simulink model "Electrical_System_2018b_obfs"  (R2019b)
settings: Solver=VariableStepAuto  StartTime=0.0  StopTime=5  RelTol=1e-3  AbsTol=1e-3  EnableMultiTasking=on
InitFcn:
  | Steady_State_Initialisation;
StopFcn:
  | %sscexplore(simlog);
  | %Logging
undefined symbols (not defined in the file): abrlhklxvp, aexgmhuedq, afmfmjnutg, afpphrjpnc, ahuxbyvruc, alarvljztt, amxnyqmnuw, aodrlwvqie, aolhmuplyq, aqpmguuqkg, auesgwirzl, aurophlnng, awamelrhru, ayfhvxflxn, azxkacuhqc, babszerikg, bawhdqanwq, bevoqecvei, bltjvqbchx, bmqsuewujl, bsmyqjfgnf, btvjbsmnve, bywgxqeadw, bziaduxaer, bzmcmdqocb, bzsvyvetat, ccsjnrbsih, cdvenygxwh, cedkrnslhx, cjheorclzs, cjrdshrtqx, ckhavyhcza, ckxewznhlz, cmrcgyiplk, conenicnws, cqkejbgjnn, csfnuwymhe, cunupkhwbh, cwzfvzuxxh, dcadmadufn, dcfponivnv, ddtrqjrhjn, dfhoxvkqas, dfrhtcwpne, dfvomcagjv, djijwylxea, dnmeqksrrm, dnzewbdkaa, dsqcykyxav, dtswwlttmm, ecumpidjtv, edegaywrct, ejjjsmnejc, eknqnehjdz, emvdetzouf, esxbqkbahr, etnkkbreiq, eunoiiiirw, ewewcuedir, fatkfxdhtc ... (+386)
libraries: fl_lib x802, ee_lib x362, fl_ps_legacy_lib x160, nesl_utility x85
(part 18 of 26)

== system Electrical_System_2018b_obfs/Redacted_1221/Redacted_7996/Redacted_7418/Redacted_4377/Redacted_6082/Redacted_2799 ==
  Redacted_14 : fl_lib/Electrical/Electrical Elements/Switch  R_closed=mmaagsrgbc Ohm  G_open=cicknjhhvm 1/Ohm  Threshold=xnzgccqlwj  i_specify=off  i_priority=None  i=hqzepkyeei A  i_nominal_specify=off  i_nominal_unit=A  i_nominal_value=vodnpbetmk  v_specify=off  v_priority=None  v=flyaivdfjk V  v_nominal_specify=off  v_nominal_unit=V  v_nominal_value=przswfymwq
      settings: SourceProductName=Simscape
  Redacted_256 : fl_lib/Electrical/Electrical Elements/Switch  R_closed=ppwmazeqls Ohm  G_open=zeylpmfzmb 1/Ohm  Threshold=xmbikwqmhm  i_specify=off  i_priority=None  i=ajinaowkbj A  i_nominal_specify=off  i_nominal_unit=A  i_nominal_value=uuuzewolju  v_specify=off  v_priority=None  v=otrqqffjwk V  v_nominal_specify=off  v_nominal_unit=V  v_nominal_value=zwxonvfcbj
      settings: SourceProductName=Simscape
  Redacted_3742 : ee_lib/Passive/Thermal/Thermal Resistor  R=xzmplidnqf K/W  T_specify=off  T_priority=None  T=zshsvjmvwr K  T_nominal_specify=off  T_nominal_unit=K  T_nominal_value=dosrqiwvts  Q_specify=off  Q_priority=None  Q=vqlgxiumlf W  Q_nominal_specify=off  Q_nominal_unit=W  Q_nominal_value=mzjjyrayck
      settings: SourceProductName=Simscape Electrical  SourceProductBaseCode=PS  InternalSimscapePortConfiguration="{\"Bottom\":[],\"Left\":[{\"id\":\"A\",\"label\":\"A\",\"type\":\"foundation.thermal.thermal\"}],\"Right\":[{\"id\":\"B\",\"label\":\"B\",\"type\":\"foundation.thermal.thermal\"}],\"Top\":[]}"
  Redacted_4034 : ee_lib/Passive/Thermal/Thermal Resistor  R=xwkozwvuwb K/W  T_specify=off  T_priority=None  T=hxycofyxfo K  T_nominal_specify=off  T_nominal_unit=K  T_nominal_value=yypnighnae  Q_specify=off  Q_priority=None  Q=mmafkkrzqa W  Q_nominal_specify=off  Q_nominal_unit=W  Q_nominal_value=whndbctdlx
      settings: SourceProductName=Simscape Electrical  SourceProductBaseCode=PS  InternalSimscapePortConfiguration="{\"Bottom\":[],\"Left\":[{\"id\":\"A\",\"label\":\"A\",\"type\":\"foundation.thermal.thermal\"}],\"Right\":[{\"id\":\"B\",\"label\":\"B\",\"type\":\"foundation.thermal.thermal\"}],\"Top\":[]}"
  Redacted_4173 : ee_lib/Semiconductors & Converters/Diode  ModelType=tulmihwegb  Vf=dqomejmcdo V  Ron=wefygixenj Ohm  Goff=cqmqzxrucq S  prmExp=eiicyzsqpu  I12=ayxwizdrlh A  V12=yndzldaqag V  IS=swswswzyjd A  ec=ortvifamwx  I1=xnvlgvzazo A  V1=cbnxrsibxn V  RS=zfzslnafvj Ohm  Tmeas=srzeczzhrz degC  N_series=cwyeowwnyg  N_parallel=rzzndodaag  Rz=tmlorzgljf Ohm  BV=fcdpsvgqfz V  C_param=oxxhjpqmkx  CJ=xdhdpetjne pF  CJ0=eopnboxorm pF  VJ=osjqldaapg V  Mgrad=sntnlkitgv  Vvec=vvvsqyjwlq V  Cvec=faidvknuuq pF  FC=nuslxbnegp  Q_param=wpcsrdqkcn  iRM=epgeeezymy A  iF=qkvtlopthh A  didt=yhywaaqkgu A/us  trr_factor=qlxokqlwik  trr=cfxrlwsbqd ns  Qrr=kjhgrlkgfn s*uA  TT=bdveackwqn ns  tau=qgwpqgtevn ns  T_param=qqwmufuloj  IS_T2=vwhbwynzbb A  I1_T2=ugrcgywvxl A  V1_T2=ofimnalxnp V  Tmeas2=efpyefnltl degC  EG_param=gkihstmgwh  EG=vfradqqcre eV  XTI_param=azeiyqzslh  XTI=jnhjlssjor  dBVdT=ozrkunrvqi V/K  Tdevice=gcqsygldcg degC  i_specify=off  i_priority=None  i=yclnvvlwuv A  i_nominal_specify=off  i_nominal_unit=A  i_nominal_value=eroqkrkcly  v_specify=off  v_priority=None  v=sctiisahnx V  v_nominal_specify=off  v_nominal_unit=V  v_nominal_value=ussldzyupi  i_capacitor_specify=off  i_capacitor_priority=None  i_capacitor=adyhzwaero A  i_capacitor_nominal_specify=off  i_capacitor_nominal_unit=A  i_capacitor_nominal_value=jlugygwjih  v_capacitor_specify=off  v_capacitor_priority=None  v_capacitor=uxlkbyjunk V  v_capacitor_nominal_specify=off  v_capacitor_nominal_unit=V  v_capacitor_nominal_value=zhqwudjppl  power_dissipated_specify=off  power_dissipated_priority=None  power_dissipated=eibromriex W  power_dissipated_nominal_specify=off  power_dissipated_nominal_unit=W  power_dissipated_nominal_value=juxdnssqlz  thermal_network_parameterization=gnvkpcxwlv  Rth=ihxwbqdmwa K/W  Rth_Foster=beymoszazb K/W  thermal_mass_parameterization=bygkjedpev  thermal_mass=rnhkfesbtn J/K  thermal_mass_Foster=zkazddkcub J/K  thermal_time_constant=iaakoydqnw s  thermal_time_constant_Foster=zdtgarfcaf s  thermal_mass_initial_temperatures=ruibdayvoi degC
      settings: SourceProductName=Simscape Electrical  InternalSimscapePortConfiguration="{\"Bottom\":[],\"Left\":[{\"id\":\"p\",\"label\":\"\",\"type\":\"foundation.electrical.electrical\"},{\"id\":\"H\",\"label\":\"H\",\"type\":\"foundation.thermal.thermal\"}],\"Right\":[{\"id\":\"n\",\"label\":\"\",\"type\":\"foundation.electrical.electrical\"}],\"Top\":[]}"
  Redacted_50 : ee_lib/Semiconductors & Converters/Diode  ModelType=tlslewfaay  Vf=peujyhvzuc V  Ron=iinywwhiso Ohm  Goff=lbfktfkkrr S  prmExp=svcvswqzek  I12=pknawufhfo A  V12=ptfuvbychd V  IS=kjqfnojdfy A  ec=flctrxnrxr  I1=ajwjiqbsyg A  V1=dxtuezywhb V  RS=ulheemthex Ohm  Tmeas=sovotrzsqy degC  N_series=kqfrjgkdxt  N_parallel=dhsfhjofpz  Rz=xnzdbvfipb Ohm  BV=kttennmtew V  C_param=trkauaxxgo  CJ=qjuoxphjll pF  CJ0=opijhorsqm pF  VJ=azylszyafb V  Mgrad=fejdgnaumo  Vvec=djwbizfuud V  Cvec=evrqxahnvx pF  FC=yrjvkpzstx  Q_param=stalshewbg  iRM=wudiijvfdv A  iF=nqxlcedqfp A  didt=lntrihncyz A/us  trr_factor=fttzoyjfdv  trr=smhwpttsrx ns  Qrr=ydzomidzbs s*uA  TT=hjyfmfchst ns  tau=enzaztgnrs ns  T_param=gtoiihraka  IS_T2=wgpmdxanuh A  I1_T2=taohkjiidl A  V1_T2=npstajglku V  Tmeas2=jdqghdjeem degC  EG_param=xydbowopwk  EG=eklyxpehqx eV  XTI_param=rffpudgvve  XTI=tirunttxyy  dBVdT=yhduoargvg V/K  Tdevice=gtbwypmaiu degC  i_specify=off  i_priority=None  i=muiumfxgrk A  i_nominal_specify=off  i_nominal_unit=A  i_nominal_value=rjdhepavsq  v_specify=off  v_priority=None  v=keyakrzcyf V  v_nominal_specify=off  v_nominal_unit=V  v_nominal_value=mwcpixjzyg  i_capacitor_specify=off  i_capacitor_priority=None  i_capacitor=qotnunkrph A  i_capacitor_nominal_specify=off  i_capacitor_nominal_unit=A  i_capacitor_nominal_value=gzchpazxzl  v_capacitor_specify=off  v_capacitor_priority=None  v_capacitor=eabcrxaphd V  v_capacitor_nominal_specify=off  v_capacitor_nominal_unit=V  v_capacitor_nominal_value=nssgdlqfnr  power_dissipated_specify=off  power_dissipated_priority=None  power_dissipated=kfsjsdylea W  power_dissipated_nominal_specify=off  power_dissipated_nominal_unit=W  power_dissipated_nominal_value=wnkkrbgvrf  thermal_network_parameterization=gawhesamhy  Rth=raeaeqquga K/W  Rth_Foster=ekchdoiazc K/W  thermal_mass_parameterization=yketfhwoay  thermal_mass=kizpyrkmou J/K  thermal_mass_Foster=noigqejeeh J/K  thermal_time_constant=klaivuzsnk s  thermal_time_constant_Foster=wylcbbwvso s  thermal_mass_initial_temperatures=meuehfpoun degC
      settings: SourceProductName=Simscape Electrical  InternalSimscapePortConfiguration="{\"Bottom\":[],\"Left\":[{\"id\":\"p\",\"label\":\"\",\"type\":\"foundation.electrical.electrical\"},{\"id\":\"H\",\"label\":\"H\",\"type\":\"foundation.thermal.thermal\"}],\"Right\":[{\"id\":\"n\",\"label\":\"\",\"type\":\"foundation.electrical.electrical\"}],\"Top\":[]}"
  Redacted_5032 : fl_lib/Electrical/Electrical Elements/Switch  R_closed=djyuvtcnkf Ohm  G_open=ejggmgjquq 1/Ohm  Threshold=rlxsobzzrp  i_specify=off  i_priority=None  i=vxccvsshfr A  i_nominal_specify=off  i_nominal_unit=A  i_nominal_value=ztoxdgmkab  v_specify=off  v_priority=None  v=mvnjgiecut V  v_nominal_specify=off  v_nominal_unit=V  v_nominal_value=fpxnpgloww
      settings: SourceProductName=Simscape
  Redacted_6997 : ee_lib/Passive/Thermal/Thermal Resistor  R=azxkacuhqc K/W  T_specify=off  T_priority=None  T=iqpeqfrrvo K  T_nominal_specify=off  T_nominal_unit=K  T_nominal_value=kewkgutqyk  Q_specify=off  Q_priority=None  Q=xgacttlsfx W  Q_nominal_specify=off  Q_nominal_unit=W  Q_nominal_value=yrupjjmulu
      settings: SourceProductName=Simscape Electrical  SourceProductBaseCode=PS  InternalSimscapePortConfiguration="{\"Bottom\":[],\"Left\":[{\"id\":\"A\",\"label\":\"A\",\"type\":\"foundation.thermal.thermal\"}],\"Right\":[{\"id\":\"B\",\"label\":\"B\",\"type\":\"foundation.thermal.thermal\"}],\"Top\":[]}"
  Redacted_7122 : ee_lib/Passive/Thermal/Thermal Resistor  R=gequosakke K/W  T_specify=off  T_priority=None  T=yveprcfpax K  T_nominal_specify=off  T_nominal_unit=K  T_nominal_value=vzsojcelwy  Q_specify=off  Q_priority=None  Q=jkflhtqewf W  Q_nominal_specify=off  Q_nominal_unit=W  Q_nominal_value=faocaagqnm
      settings: SourceProductName=Simscape Electrical  SourceProductBaseCode=PS  InternalSimscapePortConfiguration="{\"Bottom\":[],\"Left\":[{\"id\":\"A\",\"label\":\"A\",\"type\":\"foundation.thermal.thermal\"}],\"Right\":[{\"id\":\"B\",\"label\":\"B\",\"type\":\"foundation.thermal.thermal\"}],\"Top\":[]}"
  Redacted_718 : ee_lib/Semiconductors & Converters/Diode  ModelType=hzwalpwpdj  Vf=crtqorbrdf V  Ron=dtuaqqqqfe Ohm  Goff=ssskqvgjwx S  prmExp=rbylebavah  I12=gbcjlilwdj A  V12=owdgltcsjq V  IS=nrrmnrcxhi A  ec=sjfrliwacd  I1=ovljdrbuka A  V1=yrcvmuinuy V  RS=nwffojunvq Ohm  Tmeas=yszihgrhjc degC  N_series=ztkzvvauwc  N_parallel=yvkmyxeqrq  Rz=kkiditdcii Ohm  BV=eaknkoqwmh V  C_param=foimocfbtl  CJ=eiydzmpinc pF  CJ0=mcraqkkuzs pF  VJ=qixoqbkvst V  Mgrad=hddpjyowgv  Vvec=guheqtzurh V  Cvec=kdhksuhaik pF  FC=zxtvmvrhvb  Q_param=fmikkvhfee  iRM=ezawdmxmlz A  iF=gaopzjixqb A  didt=hjkdhyvheh A/us  trr_factor=zvbgvgmece  trr=ztladfgbbr ns  Qrr=ohghveggkt s*uA  TT=lfuileimpg ns  tau=toqwscqzcc ns  T_param=svdrsfxyhd  IS_T2=fcoybgbwvg A  I1_T2=aovrifrckl A  V1_T2=troutbqqfh V  Tmeas2=dvigyfmojm degC  EG_param=cxgsnvltrw  EG=roaclctwok eV  XTI_param=ytrguanjdf  XTI=oldetdbykz  dBVdT=ldyqodwnbm V/K  Tdevice=icnmseucpq degC  i_specify=off  i_priority=None  i=krxbgvsmwo A  i_nominal_specify=off  i_nominal_unit=A  i_nominal_value=gdoveeisns  v_specify=off  v_priority=None  v=blpovjuhzh V  v_nominal_specify=off  v_nominal_unit=V  v_nominal_value=qhvsoswlfe  i_capacitor_specify=off  i_capacitor_priority=None  i_capacitor=sfqremdvkr A  i_capacitor_nominal_specify=off  i_capacitor_nominal_unit=A  i_capacitor_nominal_value=rbthjluwwx  v_capacitor_specify=off  v_capacitor_priority=None  v_capacitor=gvebduyxks V  v_capacitor_nominal_specify=off  v_capacitor_nominal_unit=V  v_capacitor_nominal_value=fjsbamdorq  power_dissipated_specify=off  power_dissipated_priority=None  power_dissipated=ktvjbeqvqd W  power_dissipated_nominal_specify=off  power_dissipated_nominal_unit=W  power_dissipated_nominal_value=cyunqnofah  thermal_network_parameterization=lzdjpskjxw  Rth=tumeaafnqm K/W  Rth_Foster=kqaslzygnv K/W  thermal_mass_parameterization=jflyujjaso  thermal_mass=fpaibrkbgh J/K  thermal_mass_Foster=aldyeqrjbc J/K  thermal_time_constant=criblmxzbw s  thermal_time_constant_Foster=xulbsaulbf s  thermal_mass_initial_temperatures=glkvlbqhly degC
      settings: SourceProductName=Simscape Electrical  InternalSimscapePortConfiguration="{\"Bottom\":[],\"Left\":[{\"id\":\"p\",\"label\":\"\",\"type\":\"foundation.electrical.electrical\"},{\"id\":\"H\",\"label\":\"H\",\"type\":\"foundation.thermal.thermal\"}],\"Right\":[{\"id\":\"n\",\"label\":\"\",\"type\":\"foundation.electrical.electrical\"}],\"Top\":[]}"
  Redacted_763 : ee_lib/Semiconductors & Converters/Diode  ModelType=hdctycuzkw  Vf=tjvifnxfuv V  Ron=cnydbqsicp Ohm  Goff=ducaetsmtv S  prmExp=qgbhzhbvzj  I12=pirpzvgjxh A  V12=dkeprjwegx V  IS=elthpplyto A  ec=bvpbkohuyv  I1=oqczivjaob A  V1=pewfscyzrv V  RS=zgtelmnpgz Ohm  Tmeas=gkesqynpca degC  N_series=ihjpnnbzyc  N_parallel=lsvielbegb  Rz=ysgpebshgc Ohm  BV=atzidqevfp V  C_param=vplbhtrmxb  CJ=dvdyqfgpqq pF  CJ0=hftyrpqher pF  VJ=zurufrrrwz V  Mgrad=hvkdrxkshh  Vvec=kxomedtgot V  Cvec=xexhjpbttn pF  FC=gjtifhglrj  Q_param=mwolqugnqg  iRM=pdvcemnafx A  iF=bxrrdaeako A  didt=jneszdjouz A/us  trr_factor=bcagsmvxms  trr=ajbtpbmsxe ns  Qrr=txpyoxjdma s*uA  TT=fsnskeowqu ns  tau=cvinejynxs ns  T_param=mouvaixcwb  IS_T2=fijgahlnnp A  I1_T2=dybchooyle A  V1_T2=dfdjvdimdv V  Tmeas2=cmxztdcxjs degC  EG_param=ticuubgjcs  EG=jgngctnbnn eV  XTI_param=uttsmqjhgd  XTI=atjgiyfovh  dBVdT=inqkiimwec V/K  Tdevice=fnsyksgizi degC  i_specify=off  i_priority=None  i=gmoioopqlw A  i_nominal_specify=off  i_nominal_unit=A  i_nominal_value=xchzsubtdb  v_specify=off  v_priority=None  v=mjkywipror V  v_nominal_specify=off  v_nominal_unit=V  v_nominal_value=fkgekcnpiq  i_capacitor_specify=off  i_capacitor_priority=None  i_capacitor=icabnwcske A  i_capacitor_nominal_specify=off  i_capacitor_nominal_unit=A  i_capacitor_nominal_value=aehltcuqgt  v_capacitor_specify=off  v_capacitor_priority=None  v_capacitor=vipeafkiog V  v_capacitor_nominal_specify=off  v_capacitor_nominal_unit=V  v_capacitor_nominal_value=qnnlzbcipg  power_dissipated_specify=off  power_dissipated_priority=None  power_dissipated=hvjtajjhyi W  power_dissipated_nominal_specify=off  power_dissipated_nominal_unit=W  power_dissipated_nominal_value=nnxgpbwzip  thermal_network_parameterization=cwisxqftsu  Rth=jjddvozwen K/W  Rth_Foster=aghwyaukad K/W  thermal_mass_parameterization=atgudzouir  thermal_mass=vyptloybls J/K  thermal_mass_Foster=orlfbhuaos J/K  thermal_time_constant=crvhtflimy s  thermal_time_constant_Foster=hlgkgupwbd s  thermal_mass_initial_temperatures=frbaaqknpb degC
      settings: SourceProductName=Simscape Electrical  InternalSimscapePortConfiguration="{\"Bottom\":[],\"Left\":[{\"id\":\"p\",\"label\":\"\",\"type\":\"foundation.electrical.electrical\"},{\"id\":\"H\",\"label\":\"H\",\"type\":\"foundation.thermal.thermal\"}],\"Right\":[{\"id\":\"n\",\"label\":\"\",\"type\":\"foundation.electrical.electrical\"}],\"Top\":[]}"
  Redacted_7641 : ee_lib/Semiconductors & Converters/Diode  ModelType=jvmhhockpn  Vf=lzenknmagk V  Ron=amnubdtfvp Ohm  Goff=qakyhwvous S  prmExp=blzattelof  I12=wpanytdecq A  V12=prkwojorfo V  IS=hgjjhzphes A  ec=oewpcqfnkh  I1=vyspsvooxy A  V1=huknxinpvz V  RS=ywhdnctyml Ohm  Tmeas=blplfcoefb degC  N_series=nklolauvfh  N_parallel=ddnyewkblt  Rz=tyiiogmtyz Ohm  BV=agspwlrier V  C_param=mkgmwbzzdz  CJ=drkywxmhpg pF  CJ0=uxzofloada pF  VJ=festuymhqu V  Mgrad=zdmbswzvpp  Vvec=frqpmlhowi V  Cvec=bzftbnihgf pF  FC=nzktvefmus  Q_param=hzlsxtwhka  iRM=tobfsatnwi A  iF=xgehkjzqvu A  didt=wlzrjxtwwo A/us  trr_factor=qmfgsvlxak  trr=uaffhfasez ns  Qrr=vzqlkowmcn s*uA  TT=dtjsuxjcam ns  tau=vqppzywabh ns  T_param=vmteiodvsc  IS_T2=lyxufzuynr A  I1_T2=lbnpebfcgp A  V1_T2=fzfwfrtqhw V  Tmeas2=vcvnwnitjc degC  EG_param=knnbrzbogx  EG=ongjowqasa eV  XTI_param=ukkzrdnnfh  XTI=rtfbrnjfdp  dBVdT=iiiicbmevw V/K  Tdevice=vugruvdnuy degC  i_specify=off  i_priority=None  i=fiocoldtrl A  i_nominal_specify=off  i_nominal_unit=A  i_nominal_value=vdqgzaympr  v_specify=off  v_priority=None  v=wdejrblydg V  v_nominal_specify=off  v_nominal_unit=V  v_nominal_value=tjexfmbrlj  i_capacitor_specify=off  i_capacitor_priority=None  i_capacitor=xlhegmfnlx A  i_capacitor_nominal_specify=off  i_capacitor_nominal_unit=A  i_capacitor_nominal_value=ddhsbhtaaq  v_capacitor_specify=off  v_capacitor_priority=None  v_capacitor=kguleljzqu V  v_capacitor_nominal_specify=off  v_capacitor_nominal_unit=V  v_capacitor_nominal_value=hfthuvzvxo  power_dissipated_specify=off  power_dissipated_priority=None  power_dissipated=hkwkwlmhpj W  power_dissipated_nominal_specify=off  power_dissipated_nominal_unit=W  power_dissipated_nominal_value=orzrmogzgu  thermal_network_parameterization=ovmhndhqct  Rth=ugrkzxpapn K/W  Rth_Foster=ifwzncieyl K/W  thermal_mass_parameterization=laqtytevyp  thermal_mass=zstpknpqqu J/K  thermal_mass_Foster=yuwesjolvn J/K  thermal_time_constant=iubkltnutk s  thermal_time_constant_Foster=gunwrsxdaj s  thermal_mass_initial_temperatures=rdamugqhty degC
      settings: SourceProductName=Simscape Electrical  InternalSimscapePortConfiguration="{\"Bottom\":[],\"Left\":[{\"id\":\"p\",\"label\":\"\",\"type\":\"foundation.electrical.electrical\"},{\"id\":\"H\",\"label\":\"H\",\"type\":\"foundation.thermal.thermal\"}],\"Right\":[{\"id\":\"n\",\"label\":\"\",\"type\":\"foundation.electrical.electrical\"}],\"Top\":[]}"
  Redacted_8838 : ee_lib/Semiconductors & Converters/Diode  ModelType=cmiwftsvec  Vf=vweaeltcps V  Ron=beemewlmho Ohm  Goff=vavlbwhuvj S  prmExp=azknduoumm  I12=nyugqmmbju A  V12=bmiutjqrlm V  IS=bbpownbwtp A  ec=miqmnxjpgq  I1=sxilebsjza A  V1=esprzkqyxr V  RS=tsmillrglu Ohm  Tmeas=giaemdiozw degC  N_series=ryjyzypeuk  N_parallel=vjdnoyxwil  Rz=nxsivwbwly Ohm  BV=jycrnatugz V  C_param=czpybwxoiu  CJ=jncmqgmwwy pF  CJ0=pszifhxfry pF  VJ=muzqxdetft V  Mgrad=jontdzllgi  Vvec=fyabbwyzfg V  Cvec=hkmxdooefi pF  FC=tjdvovdkcd  Q_param=ebwmwlpwww  iRM=nggbgyzjmm A  iF=esjqdcmydr A  didt=vrwzhcrbri A/us  trr_factor=unnpuhacio  trr=rdcmaojzep ns  Qrr=icmuvztiqq s*uA  TT=xzopqsayzy ns  tau=ksscfjmwbz ns  T_param=gczfiuinnw  IS_T2=jfebpqkhnv A  I1_T2=pammjyvwmu A  V1_T2=stdljyyivk V  Tmeas2=cjmrinkojf degC  EG_param=hoqsreszcq  EG=dsrysbmqlv eV  XTI_param=iijwkinkoy  XTI=hmmsrmdojm  dBVdT=bokdbiybpf V/K  Tdevice=dacdhyyaur degC  i_specify=off  i_priority=None  i=zcbvhyriln A  i_nominal_specify=off  i_nominal_unit=A  i_nominal_value=nraaehjrvw  v_specify=off  v_priority=None  v=lcfhjijqqz V  v_nominal_specify=off  v_nominal_unit=V  v_nominal_value=xvhlohnlhz  i_capacitor_specify=off  i_capacitor_priority=None  i_capacitor=zdqctsrrvi A  i_capacitor_nominal_specify=off  i_capacitor_nominal_unit=A  i_capacitor_nominal_value=ttiqqaiibg  v_capacitor_specify=off  v_capacitor_priority=None  v_capacitor=cauazmmjzr V  v_capacitor_nominal_specify=off  v_capacitor_nominal_unit=V  v_capacitor_nominal_value=phzfwhszym  power_dissipated_specify=off  power_dissipated_priority=None  power_dissipated=qurnfxlckn W  power_dissipated_nominal_specify=off  power_dissipated_nominal_unit=W  power_dissipated_nominal_value=ymbbryiklh  thermal_network_parameterization=mmisqbvuit  Rth=glluhycnqd K/W  Rth_Foster=fkkegkuhwv K/W  thermal_mass_parameterization=tcwdmnlntr  thermal_mass=gpzqevvoni J/K  thermal_mass_Foster=opjuznapoq J/K  thermal_time_constant=hmjjgsgsya s  thermal_time_constant_Foster=rghvfyuwvo s  thermal_mass_initial_temperatures=gqkpqornjx degC
      settings: SourceProductName=Simscape Electrical  InternalSimscapePortConfiguration="{\"Bottom\":[],\"Left\":[{\"id\":\"p\",\"label\":\"\",\"type\":\"foundation.electrical.electrical\"},{\"id\":\"H\",\"label\":\"H\",\"type\":\"foundation.thermal.thermal\"}],\"Right\":[{\"id\":\"n\",\"label\":\"\",\"type\":\"foundation.electrical.electrical\"}],\"Top\":[]}"
  Redacted_5480 : PMIOPort  Side=Left
  Redacted_5609 : PMIOPort  Port=2  Side=Left
  Redacted_8475 : PMIOPort  Port=3  Side=Left
  Redacted_2850 : PMIOPort  Port=4  Side=Right
  Redacted_1993 : PMIOPort  Port=5  Side=Right
  Redacted_7871 : PMIOPort  Port=6  Side=Right
  Redacted_7603 : PMIOPort  Port=7  Side=Left
  Redacted_3441 : PMIOPort  Port=8  Side=Right
  connections:
  Redacted_8838/LConn1 -- Redacted_5609/RConn1 -- Redacted_718/RConn1
  Redacted_8838/RConn1 -- Redacted_256/LConn1 -- Redacted_718/LConn1
  Redacted_3742/LConn1 -- Redacted_763/LConn2 -- Redacted_50/LConn2
  Redacted_2850/RConn1 -- Redacted_5032/RConn2
  Redacted_50/LConn1 -- Redacted_5032/LConn1 -- Redacted_763/RConn1
  Redacted_763/LConn1 -- Redacted_5480/RConn1 -- Redacted_50/RConn1
  Redacted_7122/RConn1 -- Redacted_4034/RConn1 -- Redacted_6997/LConn1 -- Redacted_3742/RConn1
  Redacted_7641/LConn1 -- Redacted_8475/RConn1 -- Redacted_4173/RConn1
  Redacted_7871/RConn1 -- Redacted_14/RConn2
  Redacted_3441/RConn1 -- Redacted_14/RConn1 -- Redacted_256/RConn1 -- Redacted_5032/RConn1
  Redacted_1993/RConn1 -- Redacted_256/RConn2
  Redacted_4173/LConn1 -- Redacted_14/LConn1 -- Redacted_7641/RConn1
  Redacted_4173/LConn2 -- Redacted_4034/LConn1 -- Redacted_7641/LConn2
  Redacted_6997/RConn1 -- Redacted_7603/RConn1
  Redacted_8838/LConn2 -- Redacted_718/LConn2 -- Redacted_7122/LConn1

== system Electrical_System_2018b_obfs/Redacted_1221/Redacted_7996/Redacted_7418/Redacted_4377/Redacted_6082/Redacted_2927 ==
  Neutral_Negative : Subsystem  VariantControl=Variant1
  Positive_Neutral : Subsystem  VariantControl=Variant3
  Redacted_9228 : Subsystem  VariantControl=Variant2
  Redacted_7425 : PMIOPort  Side=Left
  Redacted_110 : PMIOPort  Port=2  Side=Left
  Redacted_9932 : PMIOPort  Port=3  Side=Left
  Redacted_5448 : PMIOPort  Port=4  Side=Right
  Redacted_18 : PMIOPort  Port=5  Side=Right

== system Electrical_System_2018b_obfs/Redacted_1221/Redacted_7996/Redacted_7418/Redacted_4377/Redacted_6082/Redacted_3086 ==
  Neutral_Negative : Subsystem  VariantControl=Variant1
  Positive_Neutral : Subsystem  VariantControl=Variant3
  Redacted_7741 : Subsystem  VariantControl=Variant2
  Redacted_6054 : PMIOPort  Side=Left
  Redacted_5626 : PMIOPort  Port=2  Side=Left
  Redacted_6271 : PMIOPort  Port=3  Side=Left
  Redacted_2564 : PMIOPort  Port=4  Side=Right
  Redacted_7933 : PMIOPort  Port=5  Side=Right

== system Electrical_System_2018b_obfs/Redacted_1221/Redacted_7996/Redacted_7418/Redacted_4377/Redacted_6082/Redacted_3181 ==
  Redacted_1351 : ee_lib/Semiconductors & Converters/Diode  ModelType=seeuamuunc  Vf=tjetfrvgds V  Ron=tkwkxekvdq Ohm  Goff=xzxgjjbiog S  prmExp=tjyqkmyyzz  I12=vfldstogen A  V12=aavwtmhros V  IS=bjqywamhpj A  ec=kdkykdyevk  I1=zmbpaboecy A  V1=udzpdlacpc V  RS=jxlihmcwve Ohm  Tmeas=yyfgspfgbd degC  N_series=zsfxqjbunr  N_parallel=fgwiengsno  Rz=avicgvmlgk Ohm  BV=okerteawrl V  C_param=wbkqkuwogq  CJ=wjeiksybxp pF  CJ0=bhyyzfyxjp pF  VJ=baqqiwdxpe V  Mgrad=ijgrywoabh  Vvec=hkmchzqwjs V  Cvec=boveevrcen pF  FC=zabwgjpoen  Q_param=eawnjzzyvy  iRM=kamsrqwhqk A  iF=gaslkmmfnx A  didt=ntyglgoooi A/us  trr_factor=sysuzqibag  trr=yinnobosjz ns  Qrr=jaajtcswbs s*uA  TT=nsneizmgzk ns  tau=gvehbplkpv ns  T_param=rmggrjeyry  IS_T2=bosnjnhbqx A  I1_T2=sevxlylkmu A  V1_T2=kuctfzdxpm V  Tmeas2=xsehdofiyo degC  EG_param=oeofywqxdk  EG=uifethuxrb eV  XTI_param=wtzpwykpco  XTI=jqlhgbjlia  dBVdT=bvciagvedp V/K  Tdevice=wqvmrlhfms degC  i_specify=off  i_priority=None  i=iibbfecdkw A  i_nominal_specify=off  i_nominal_unit=A  i_nominal_value=rqcvvpbxgl  v_specify=off  v_priority=None  v=ozhvdnmemj V  v_nominal_specify=off  v_nominal_unit=V  v_nominal_value=rgrbkwjmip  i_capacitor_specify=off  i_capacitor_priority=None  i_capacitor=hbcekzmgcv A  i_capacitor_nominal_specify=off  i_capacitor_nominal_unit=A  i_capacitor_nominal_value=hspgnyvvck  v_capacitor_specify=off  v_capacitor_priority=None  v_capacitor=ekhmskymom V  v_capacitor_nominal_specify=off  v_capacitor_nominal_unit=V  v_capacitor_nominal_value=kxjlgmioqp  power_dissipated_specify=off  power_dissipated_priority=None  power_dissipated=edojgqvblt W  power_dissipated_nominal_specify=off  power_dissipated_nominal_unit=W  power_dissipated_nominal_value=tsdphnszae  thermal_network_parameterization=asyzzvkyhi  Rth=lywppooubx K/W  Rth_Foster=vecederauj K/W  thermal_mass_parameterization=fsmsxwodxt  thermal_mass=udhbpbteyl J/K  thermal_mass_Foster=kcaieczpfc J/K  thermal_time_constant=qqooakurgg s  thermal_time_constant_Foster=zxqadwzazc s  thermal_mass_initial_temperatures=ljlpeezqox degC
      settings: SourceProductName=Simscape Electrical  InternalSimscapePortConfiguration="{\"Bottom\":[],\"Left\":[{\"id\":\"p\",\"label\":\"\",\"type\":\"foundation.electrical.electrical\"},{\"id\":\"H\",\"label\":\"H\",\"type\":\"foundation.thermal.thermal\"}],\"Right\":[{\"id\":\"n\",\"label\":\"\",\"type\":\"foundation.electrical.electrical\"}],\"Top\":[]}"
  Redacted_3158 : fl_lib/Electrical/Electrical Elements/Switch  R_closed=hwmyltiiqs Ohm  G_open=oageffilii 1/Ohm  Threshold=llxzcykggr  i_specify=off  i_priority=None  i=towpqqbrgr A  i_nominal_specify=off  i_nominal_unit=A  i_nominal_value=yhnwwkhofb  v_specify=off  v_priority=None  v=qsxecyuspm V  v_nominal_specify=off  v_nominal_unit=V  v_nominal_value=iycquvnywo
      settings: SourceProductName=Simscape
  Redacted_3931 : ee_lib/Semiconductors & Converters/Diode  ModelType=tqxwxbyope  Vf=msvpzzkeba V  Ron=fwkchzqblf Ohm  Goff=svlnqffeyd S  prmExp=mlctstspcp  I12=bbyevmnspz A  V12=uvkidbyuvs V  IS=lpydrxcezd A  ec=qsufrycozn  I1=lepjzvxqxl A  V1=ipknupmupx V  RS=bzinarmuqq Ohm  Tmeas=rkwjjzfkwq degC  N_series=imzifmjoup  N_parallel=wbyltkjjsq  Rz=bisuniwcvj Ohm  BV=jgybmonlsf V  C_param=hbgjuibrwj  CJ=gqvyumecto pF  CJ0=ibsphiesxm pF  VJ=bijqmoevpa V  Mgrad=mubmyiximf  Vvec=byiivkqhni V  Cvec=aoibtvakqs pF  FC=copuhvmvyb  Q_param=bflbuobaow  iRM=zldaqxybvj A  iF=ytnymxtjly A  didt=idoehkwwtj A/us  trr_factor=ebltoywncm  trr=fygpxetjfj ns  Qrr=uimcleybda s*uA  TT=krndejyjuq ns  tau=hukxqqjqto ns  T_param=elgqdsktyc  IS_T2=zbjbtcnzao A  I1_T2=hipcbswwjs A  V1_T2=dsoyluttfa V  Tmeas2=fbupxbajck degC  EG_param=mvsexujbus  EG=xiyujyeecx eV  XTI_param=krdlbkxuyu  XTI=xewpkszqxo  dBVdT=ibvfxirjgx V/K  Tdevice=rknouiddqv degC  i_specify=off  i_priority=None  i=ecenxenwrc A  i_nominal_specify=off  i_nominal_unit=A  i_nominal_value=fxilzhobes  v_specify=off  v_priority=None  v=hrmiwxfjsj V  v_nominal_specify=off  v_nominal_unit=V  v_nominal_value=emarxszixz  i_capacitor_specify=off  i_capacitor_priority=None  i_capacitor=febrtrnqtb A  i_capacitor_nominal_specify=off  i_capacitor_nominal_unit=A  i_capacitor_nominal_value=jccfenurhb  v_capacitor_specify=off  v_capacitor_priority=None  v_capacitor=umlvqkknjw V  v_capacitor_nominal_specify=off  v_capacitor_nominal_unit=V  v_capacitor_nominal_value=gghvoucqhq  power_dissipated_specify=off  power_dissipated_priority=None  power_dissipated=amzqicgaia W  power_dissipated_nominal_specify=off  power_dissipated_nominal_unit=W  power_dissipated_nominal_value=oymruehjkf  thermal_network_parameterization=jpsxuylylh  Rth=uehbhvrzjt K/W  Rth_Foster=tejtqvzged K/W  thermal_mass_parameterization=btxpxztosi  thermal_mass=gxhkmzniwp J/K  thermal_mass_Foster=vdvluvqrgk J/K  thermal_time_constant=idwezoowwk s  thermal_time_constant_Foster=iskjzblkee s  thermal_mass_initial_temperatures=rnchfspvkh degC
      settings: SourceProductName=Simscape Electrical  InternalSimscapePortConfiguration="{\"Bottom\":[],\"Left\":[{\"id\":\"p\",\"label\":\"\",\"type\":\"foundation.electrical.electrical\"},{\"id\":\"H\",\"label\":\"H\",\"type\":\"foundation.thermal.thermal\"}],\"Right\":[{\"id\":\"n\",\"label\":\"\",\"type\":\"foundation.electrical.electrical\"}],\"Top\":[]}"
  Redacted_4404 : ee_lib/Passive/Thermal/Thermal Resistor  R=xexuroemqo K/W  T_specify=off  T_priority=None  T=xnbryopseg K  T_nominal_specify=off  T_nominal_unit=K  T_nominal_value=kdpocicxnp  Q_specify=off  Q_priority=None  Q=hdqjdfbsma W  Q_nominal_specify=off  Q_nominal_unit=W  Q_nominal_value=udkikzuzos
      settings: SourceProductName=Simscape Electrical  SourceProductBaseCode=PS  InternalSimscapePortConfiguration="{\"Bottom\":[],\"Left\":[{\"id\":\"A\",\"label\":\"A\",\"type\":\"foundation.thermal.thermal\"}],\"Right\":[{\"id\":\"B\",\"label\":\"B\",\"type\":\"foundation.thermal.thermal\"}],\"Top\":[]}"
  Redacted_6446 : ee_lib/Passive/Thermal/Thermal Resistor  R=hwqngtoeuw K/W  T_specify=off  T_priority=None  T=hsoozjtrph K  T_nominal_specify=off  T_nominal_unit=K  T_nominal_value=dxhlmwnjse  Q_specify=off  Q_priority=None  Q=nagsetwglx W  Q_nominal_specify=off  Q_nominal_unit=W  Q_nominal_value=cxhyvgnbrj
      settings: SourceProductName=Simscape Electrical  SourceProductBaseCode=PS  InternalSimscapePortConfiguration="{\"Bottom\":[],\"Left\":[{\"id\":\"A\",\"label\":\"A\",\"type\":\"foundation.thermal.thermal\"}],\"Right\":[{\"id\":\"B\",\"label\":\"B\",\"type\":\"foundation.thermal.thermal\"}],\"Top\":[]}"
  Redacted_9048 : ee_lib/Passive/Thermal/Thermal Resistor  R=zjtbpuzrue K/W  T_specify=off  T_priority=None  T=etnkkbreiq K  T_nominal_specify=off  T_nominal_unit=K  T_nominal_value=kahcrnokjt  Q_specify=off  Q_priority=None  Q=lionqndkkr W  Q_nominal_specify=off  Q_nominal_unit=W  Q_nominal_value=rkfkvndftj
      settings: SourceProductName=Simscape Electrical  SourceProductBaseCode=PS  InternalSimscapePortConfiguration="{\"Bottom\":[],\"Left\":[{\"id\":\"A\",\"label\":\"A\",\"type\":\"foundation.thermal.thermal\"}],\"Right\":[{\"id\":\"B\",\"label\":\"B\",\"type\":\"foundation.thermal.thermal\"}],\"Top\":[]}"
  Redacted_9733 : fl_lib/Electrical/Electrical Elements/Switch  R_closed=ovhcdwdqkf Ohm  G_open=owpytlrcdh 1/Ohm  Threshold=yzytgmynyn  i_specify=off  i_priority=None  i=owtxshledt A  i_nominal_specify=off  i_nominal_unit=A  i_nominal_value=nybtewbswk  v_specify=off  v_priority=None  v=kpnujakptf V  v_nominal_specify=off  v_nominal_unit=V  v_nominal_value=jucrzeyoqp
      settings: SourceProductName=Simscape
  Redacted_2911 : PMIOPort  Side=Left
  Redacted_7251 : PMIOPort  Port=2  Side=Left
  Redacted_7245 : PMIOPort  Port=3  Side=Right
  Redacted_1415 : PMIOPort  Port=4  Side=Right
  Redacted_532 : PMIOPort  Port=5  Side=Left
  Redacted_2658 : PMIOPort  Port=6  Side=Right
  connections:
  Redacted_3931/LConn1 -- Redacted_7251/RConn1
  Redacted_3931/RConn1 -- Redacted_3158/LConn1
  Redacted_1351/LConn2 -- Redacted_6446/LConn1
  Redacted_7245/RConn1 -- Redacted_9733/RConn2
  Redacted_1351/LConn1 -- Redacted_9733/LConn1
  Redacted_2911/RConn1 -- Redacted_1351/RConn1
  Redacted_4404/RConn1 -- Redacted_9048/LConn1 -- Redacted_6446/RConn1
  Redacted_2658/RConn1 -- Redacted_3158/RConn1 -- Redacted_9733/RConn1
  Redacted_1415/RConn1 -- Redacted_3158/RConn2
  Redacted_9048/RConn1 -- Redacted_532/RConn1
  Redacted_3931/LConn2 -- Redacted_4404/LConn1

== system Electrical_System_2018b_obfs/Redacted_1221/Redacted_7996/Redacted_7418/Redacted_4377/Redacted_6082/Redacted_3818 ==
  Neutral_Negative : Subsystem  VariantControl=Variant1
  Positive_Neutral : Subsystem  VariantControl=Variant3
  Redacted_7647 : Subsystem  VariantControl=Variant2
  Redacted_558 : PMIOPort  Side=Left
  Redacted_9353 : PMIOPort  Port=2  Side=Left
  Redacted_2763 : PMIOPort  Port=3  Side=Left
  Redacted_5509 : PMIOPort  Port=4  Side=Right
  Redacted_3127 : PMIOPort  Port=5  Side=Right

== system Electrical_System_2018b_obfs/Redacted_1221/Redacted_7996/Redacted_7418/Redacted_4377/Redacted_6082/Redacted_4174 ==
  Neutral_Negative : Subsystem  VariantControl=Variant1
  Positive_Neutral : Subsystem  VariantControl=Variant3
  Redacted_8370 : Subsystem  VariantControl=Variant2
  Redacted_9679 : PMIOPort  Side=Left
  Redacted_9878 : PMIOPort  Port=2  Side=Left
  Redacted_224 : PMIOPort  Port=3  Side=Left
  Redacted_5953 : PMIOPort  Port=4  Side=Right
  Redacted_7639 : PMIOPort  Port=5  Side=Right

== system Electrical_System_2018b_obfs/Redacted_1221/Redacted_7996/Redacted_7418/Redacted_4377/Redacted_6082/Redacted_4278 ==
  Neutral_Negative : Subsystem  VariantControl=Variant1
  Positive_Neutral : Subsystem  VariantControl=Variant3
  Redacted_1592 : Subsystem  VariantControl=Variant2
  Redacted_1495 : PMIOPort  Side=Left
  Redacted_2064 : PMIOPort  Port=2  Side=Left
  Redacted_9467 : PMIOPort  Port=3  Side=Left
  Redacted_1543 : PMIOPort  Port=4  Side=Right
  Redacted_9491 : PMIOPort  Port=5  Side=Right

== system Electrical_System_2018b_obfs/Redacted_1221/Redacted_7996/Redacted_7418/Redacted_4377/Redacted_6082/Redacted_4288 ==
  Redacted_1420 : ee_lib/Passive/Thermal/Thermal Resistor  R=csfnuwymhe K/W  T_specify=off  T_priority=None  T=dfrhtcwpne K  T_nominal_specify=off  T_nominal_unit=K  T_nominal_value=undcbzrngw  Q_specify=off  Q_priority=None  Q=qyyvrynvtf W  Q_nominal_specify=off  Q_nominal_unit=W  Q_nominal_value=fykywgxewt
      settings: SourceProductName=Simscape Electrical  SourceProductBaseCode=PS  InternalSimscapePortConfiguration="{\"Bottom\":[],\"Left\":[{\"id\":\"A\",\"label\":\"A\",\"type\":\"foundation.thermal.thermal\"}],\"Right\":[{\"id\":\"B\",\"label\":\"B\",\"type\":\"foundation.thermal.thermal\"}],\"Top\":[]}"
  Redacted_3053 : ee_lib/Passive/Thermal/Thermal Resistor  R=feuklzgtpa K/W  T_specify=off  T_priority=None  T=qwktvjvfys K  T_nominal_specify=off  T_nominal_unit=K  T_nominal_value=arolkdlhmd  Q_specify=off  Q_priority=None  Q=djhelqxest W  Q_nominal_specify=off  Q_nominal_unit=W  Q_nominal_value=dkqmeratgj
      settings: SourceProductName=Simscape Electrical  SourceProductBaseCode=PS  InternalSimscapePortConfiguration="{\"Bottom\":[],\"Left\":[{\"id\":\"A\",\"label\":\"A\",\"type\":\"foundation.thermal.thermal\"}],\"Right\":[{\"id\":\"B\",\"label\":\"B\",\"type\":\"foundation.thermal.thermal\"}],\"Top\":[]}"
  Redacted_5187 : fl_lib/Electrical/Electrical Elements/Switch  R_closed=iidrcmgruo Ohm  G_open=cwflxapbrg 1/Ohm  Threshold=wtaszsnldr  i_specify=off  i_priority=None  i=cfjwrmlajq A  i_nominal_specify=off  i_nominal_unit=A  i_nominal_value=qzidrdxbsm  v_specify=off  v_priority=None  v=hrbzqwpexo V  v_nominal_specify=off  v_nominal_unit=V  v_nominal_value=oarcvjnccc
      settings: SourceProductName=Simscape
  Redacted_5716 : fl_lib/Electrical/Electrical Elements/Switch  R_closed=krkbgwsxlo Ohm  G_open=nwjalbnmwo 1/Ohm  Threshold=wlnjmfizfx  i_specify=off  i_priority=None  i=xtkvqzsayg A  i_nominal_specify=off  i_nominal_unit=A  i_nominal_value=nzimhpxyaj  v_specify=off  v_priority=None  v=dcozybqfae V  v_nominal_specify=off  v_nominal_unit=V  v_nominal_value=cwsubwwopk
      settings: SourceProductName=Simscape
  Redacted_631 : ee_lib/Semiconductors & Converters/Diode  ModelType=kwymznercn  Vf=bzeobnkmpp V  Ron=ogzcuqezum Ohm  Goff=hboakganul S  prmExp=tspwxvmtix  I12=vzhmfidnsx A  V12=lzcdoaedsk V  IS=lxuhqgdzyf A  ec=lgmvvpmtfb  I1=wubgixerlf A  V1=ghqnutyshn V  RS=yfueffmaxl Ohm  Tmeas=ydajfmxqbx degC  N_series=yivbhcvoir  N_parallel=htzntkphxa  Rz=qvvvhxwbpi Ohm  BV=ymjzdmieqs V  C_param=msvgljfcfw  CJ=zsrrieohii pF  CJ0=tuthjrqdnh pF  VJ=nycerhqgyj V  Mgrad=qvizemveid  Vvec=qlenbgnmqk V  Cvec=bligwbbtgp pF  FC=roozurrocc  Q_param=xkglsmbrbh  iRM=qahgubavsm A  iF=pufyexdedl A  didt=isjydruslg A/us  trr_factor=dffqwpsdyp  trr=anfkerbzue ns  Qrr=deomtvnwwe s*uA  TT=lrekwszonl ns  tau=iyastrgkxi ns  T_param=kjwuhembzs  IS_T2=mmckjlxiwy A  I1_T2=llsygjllnm A  V1_T2=ebzpqvnskm V  Tmeas2=dgihdwdint degC  EG_param=vfglbqzjmq  EG=vnjpxdvxmw eV  XTI_param=uocmdbuhnh  XTI=mybmalgdic  dBVdT=fpdhcmbsix V/K  Tdevice=fyegxrufcw degC  i_specify=off  i_priority=None  i=lkokslneyy A  i_nominal_specify=off  i_nominal_unit=A  i_nominal_value=hoeahmmfuu  v_specify=off  v_priority=None  v=jwstxjltpj V  v_nominal_specify=off  v_nominal_unit=V  v_nominal_value=vzfhxnllbc  i_capacitor_specify=off  i_capacitor_priority=None  i_capacitor=myvfxzqlck A  i_capacitor_nominal_specify=off  i_capacitor_nominal_unit=A  i_capacitor_nominal_value=roqvolylnm  v_capacitor_specify=off  v_capacitor_priority=None  v_capacitor=gptluhsrhz V  v_capacitor_nominal_specify=off  v_capacitor_nominal_unit=V  v_capacitor_nominal_value=alzbeepcwm  power_dissipated_specify=off  power_dissipated_priority=None  power_dissipated=uijibnuhos W  power_dissipated_nominal_specify=off  power_dissipated_nominal_unit=W  power_dissipated_nominal_value=lbddeeurpg  thermal_network_parameterization=frunhdzzzq  Rth=ipffswvaig K/W  Rth_Foster=tpgcjeuyzq K/W  thermal_mass_parameterization=jwlodfpkvm  thermal_mass=ehnyrrnqzl J/K  thermal_mass_Foster=unmbisyvtm J/K  thermal_time_constant=oypiywoukf s  thermal_time_constant_Foster=xnmvgxpcww s  thermal_mass_initial_temperatures=zwgjhousxc degC
      settings: SourceProductName=Simscape Electrical  InternalSimscapePortConfiguration="{\"Bottom\":[],\"Left\":[{\"id\":\"p\",\"label\":\"\",\"type\":\"foundation.electrical.electrical\"},{\"id\":\"H\",\"label\":\"H\",\"type\":\"foundation.thermal.thermal\"}],\"Right\":[{\"id\":\"n\",\"label\":\"\",\"type\":\"foundation.electrical.electrical\"}],\"Top\":[]}"
  Redacted_6763 : ee_lib/Semiconductors & Converters/Diode  ModelType=clgixcnwoc  Vf=ftpzcjmppy V  Ron=dbcidwevvn Ohm  Goff=yhrmcwzgue S  prmExp=aisizesfzq  I12=lacnnvocyc A  V12=pbpbsjubgs V  IS=xamdbquppu A  ec=eeecjfdprz  I1=yjljdcozpv A  V1=ffbopghzjw V  RS=wcqnbvzzev Ohm  Tmeas=kbuiibngbo degC  N_series=qqlilfwukw  N_parallel=fxbsiddyro  Rz=dodwndnmkr Ohm  BV=liehghwjmv V  C_param=vktsvahwle  CJ=fhntaxxfft pF  CJ0=qumaznckyu pF  VJ=xpoblmifuo V  Mgrad=ocusdggsnv  Vvec=seffqhedpz V  Cvec=ohcmggolrz pF  FC=yxsxrkinug  Q_param=bvzohlmuww  iRM=xicczpmsfr A  iF=rkcnntyhvb A  didt=vtudfiaipt A/us  trr_factor=rqvaooxfvk  trr=tvwihwyihb ns  Qrr=kulozvhoez s*uA  TT=nitkbtqglp ns  tau=ubqxhynwqh ns  T_param=igxsyorppi  IS_T2=mqvbxmpxvg A  I1_T2=armqecybmn A  V1_T2=muvfioogix V  Tmeas2=ppsjgixytg degC  EG_param=xjxvdcpxwh  EG=agihhvisij eV  XTI_param=yuocwdmjkw  XTI=xoszctygzp  dBVdT=uoohrvaigf V/K  Tdevice=qhfnbogqqg degC  i_specify=off  i_priority=None  i=qtedmgmqsm A  i_nominal_specify=off  i_nominal_unit=A  i_nominal_value=mqkthilpvy  v_specify=off  v_priority=None  v=itpbbundcp V  v_nominal_specify=off  v_nominal_unit=V  v_nominal_value=ykhzflpcnx  i_capacitor_specify=off  i_capacitor_priority=None  i_capacitor=uryfeeajta A  i_capacitor_nominal_specify=off  i_capacitor_nominal_unit=A  i_capacitor_nominal_value=ftxeerromd  v_capacitor_specify=off  v_capacitor_priority=None  v_capacitor=hddhodbyvb V  v_capacitor_nominal_specify=off  v_capacitor_nominal_unit=V  v_capacitor_nominal_value=yzdcvmjrfh  power_dissipated_specify=off  power_dissipated_priority=None  power_dissipated=aaxygncreu W  power_dissipated_nominal_specify=off  power_dissipated_nominal_unit=W  power_dissipated_nominal_value=xuxnetzqve  thermal_network_parameterization=zrkkuhurzb  Rth=odsbqwesbo K/W  Rth_Foster=ibbukupzba K/W  thermal_mass_parameterization=laqxzbiuja  thermal_mass=jqetfysksy J/K  thermal_mass_Foster=rleuvpzybd J/K  thermal_time_constant=vfwhldlplc s  thermal_time_constant_Foster=sredobdxmn s  thermal_mass_initial_temperatures=gkskoiqoer degC
      settings: SourceProductName=Simscape Electrical  InternalSimscapePortConfiguration="{\"Bottom\":[],\"Left\":[{\"id\":\"p\",\"label\":\"\",\"type\":\"foundation.electrical.electrical\"},{\"id\":\"H\",\"label\":\"H\",\"type\":\"foundation.thermal.thermal\"}],\"Right\":[{\"id\":\"n\",\"label\":\"\",\"type\":\"foundation.electrical.electrical\"}],\"Top\":[]}"
  Redacted_938 : ee_lib/Passive/Thermal/Thermal Resistor  R=virfgdrnfz K/W  T_specify=off  T_priority=None  T=alarvljztt K  T_nominal_specify=off  T_nominal_unit=K  T_nominal_value=joqgdgroxe  Q_specify=off  Q_priority=None  Q=kaqfzywiqi W  Q_nominal_specify=off  Q_nominal_unit=W  Q_nominal_value=zlmidgadwg
      settings: SourceProductName=Simscape Electrical  SourceProductBaseCode=PS  InternalSimscapePortConfiguration="{\"Bottom\":[],\"Left\":[{\"id\":\"A\",\"label\":\"A\",\"type\":\"foundation.thermal.thermal\"}],\"Right\":[{\"id\":\"B\",\"label\":\"B\",\"type\":\"foundation.thermal.thermal\"}],\"Top\":[]}"
  Redacted_2382 : PMIOPort  Side=Left
  Redacted_435 : PMIOPort  Port=2  Side=Left
  Redacted_3794 : PMIOPort  Port=3  Side=Right
  Redacted_28 : PMIOPort  Port=4  Side=Right
  Redacted_1383 : PMIOPort  Port=5  Side=Left
  Redacted_1778 : PMIOPort  Port=6  Side=Right
  connections:
  Redacted_6763/LConn1 -- Redacted_435/RConn1
  Redacted_6763/RConn1 -- Redacted_5716/LConn1
  Redacted_631/LConn2 -- Redacted_938/LConn1
  Redacted_3794/RConn1 -- Redacted_5187/RConn2
  Redacted_631/LConn1 -- Redacted_5187/LConn1
  Redacted_2382/RConn1 -- Redacted_631/RConn1
  Redacted_3053/RConn1 -- Redacted_1420/LConn1 -- Redacted_938/RConn1
  Redacted_1778/RConn1 -- Redacted_5716/RConn1 -- Redacted_5187/RConn1
  Redacted_28/RConn1 -- Redacted_5716/RConn2
  Redacted_1420/RConn1 -- Redacted_1383/RConn1
  Redacted_6763/LConn2 -- Redacted_3053/LConn1

== system Electrical_System_2018b_obfs/Redacted_1221/Redacted_7996/Redacted_7418/Redacted_4377/Redacted_6082/Redacted_4413 ==
  Neutral_Negative : Subsystem  VariantControl=Variant1
  Positive_Neutral : Subsystem  VariantControl=Variant3
  Redacted_6190 : Subsystem  VariantControl=Variant2
  Redacted_9976 : PMIOPort  Side=Left
  Redacted_5180 : PMIOPort  Port=2  Side=Left
  Redacted_6712 : PMIOPort  Port=3  Side=Left
  Redacted_6595 : PMIOPort  Port=4  Side=Right
  Redacted_8408 : PMIOPort  Port=5  Side=Right

== system Electrical_System_2018b_obfs/Redacted_1221/Redacted_7996/Redacted_7418/Redacted_4377/Redacted_6082/Redacted_4712 ==
  Redacted_2183 : ee_lib/Passive/Thermal/Thermal Resistor  R=uwrxzutslg K/W  T_specify=off  T_priority=None  T=pajgcmnuxp K  T_nominal_specify=off  T_nominal_unit=K  T_nominal_value=oprwgenfni  Q_specify=off  Q_priority=None  Q=vnctjcpbal W  Q_nominal_specify=off  Q_nominal_unit=W  Q_nominal_value=rnairkbzzr
      settings: SourceProductName=Simscape Electrical  SourceProductBaseCode=PS  InternalSimscapePortConfiguration="{\"Bottom\":[],\"Left\":[{\"id\":\"A\",\"label\":\"A\",\"type\":\"foundation.thermal.thermal\"}],\"Right\":[{\"id\":\"B\",\"label\":\"B\",\"type\":\"foundation.thermal.thermal\"}],\"Top\":[]}"
  Redacted_2562 : fl_lib/Electrical/Electrical Elements/Switch  R_closed=vkroixkmza Ohm  G_open=aclkmnqnqn 1/Ohm  Threshold=mqphwqpqtk  i_specify=off  i_priority=None  i=wqsnzdmaqu A  i_nominal_specify=off  i_nominal_unit=A  i_nominal_value=jdsbnyvvrn  v_specify=off  v_priority=None  v=mtgnvxvoef V  v_nominal_specify=off  v_nominal_unit=V  v_nominal_value=xpdcqtwjkq
      settings: SourceProductName=Simscape
  Redacted_4076 : fl_lib/Electrical/Electrical Elements/Switch  R_closed=njwxpudroe Ohm  G_open=unopnvzees 1/Ohm  Threshold=vnjqsgeems  i_specify=off  i_priority=None  i=tvyggmthfk A  i_nominal_specify=off  i_nominal_unit=A  i_nominal_value=fudhxnvthp  v_specify=off  v_priority=None  v=blecxtmuzk V  v_nominal_specify=off  v_nominal_unit=V  v_nominal_value=mxbomhtqdj
      settings: SourceProductName=Simscape
  Redacted_4934 : ee_lib/Passive/Thermal/Thermal Resistor  R=qtaxfrwwfd K/W  T_specify=off  T_priority=None  T=jbhnvsqxgq K  T_nominal_specify=off  T_nominal_unit=K  T_nominal_value=wqgbotzlrn  Q_specify=off  Q_priority=None  Q=oiubxlneqr W  Q_nominal_specify=off  Q_nominal_unit=W  Q_nominal_value=qhrxutyvpm
      settings: SourceProductName=Simscape Electrical  SourceProductBaseCode=PS  InternalSimscapePortConfiguration="{\"Bottom\":[],\"Left\":[{\"id\":\"A\",\"label\":\"A\",\"type\":\"foundation.thermal.thermal\"}],\"Right\":[{\"id\":\"B\",\"label\":\"B\",\"type\":\"foundation.thermal.thermal\"}],\"Top\":[]}"
  Redacted_6160 : ee_lib/Semiconductors & Converters/Diode  ModelType=wxghzbmewo  Vf=incyrzxxzf V  Ron=bufhejqsgj Ohm  Goff=bzmmwltpda S  prmExp=oyufyuxxul  I12=zqevqndhvr A  V12=ntgabtemlm V  IS=esogqbbpag A  ec=mhmrjglsyl  I1=baysikteys A  V1=jddnlczanv V  RS=xilzloxftw Ohm  Tmeas=hshgidoefp degC  N_series=tvwlqlappu  N_parallel=ynyhscmuqe  Rz=biacdhtehh Ohm  BV=vcztypyixs V  C_param=ymjusrygft  CJ=nzixmodzqw pF  CJ0=rmyzhcbopm pF  VJ=texbhuncud V  Mgrad=tkridumood  Vvec=jbuxjwgifj V  Cvec=yijsdqpcdn pF  FC=joqholwqmr  Q_param=iqextqebao  iRM=oosasuiphy A  iF=aqxfnvhdsh A  didt=iuypvkuhmr A/us  trr_factor=dqnmklrpvy  trr=rwbczlghkl ns  Qrr=ashruozjcw s*uA  TT=bxoqkmimcn ns  tau=upkecktgtn ns  T_param=whgrtbtgkt  IS_T2=ytmdinuaho A  I1_T2=poblvhcxkr A  V1_T2=hnwmatqgpq V  Tmeas2=jrgnekkvfk degC  EG_param=tblraoxtej  EG=timwdxryfu eV  XTI_param=btzoraanbl  XTI=wflfvuhjxp  dBVdT=xvknpvwxts V/K  Tdevice=gmzsticnnk degC  i_specify=off  i_priority=None  i=qefslitdry A  i_nominal_specify=off  i_nominal_unit=A  i_nominal_value=qcpugyhbqw  v_specify=off  v_priority=None  v=gggiokbjmg V  v_nominal_specify=off  v_nominal_unit=V  v_nominal_value=scytvwxumi  i_capacitor_specify=off  i_capacitor_priority=None  i_capacitor=qsjysvanbz A  i_capacitor_nominal_specify=off  i_capacitor_nominal_unit=A  i_capacitor_nominal_value=pewfqtvxxi  v_capacitor_specify=off  v_capacitor_priority=None  v_capacitor=bwoefqwwqs V  v_capacitor_nominal_specify=off  v_capacitor_nominal_unit=V  v_capacitor_nominal_value=mkonfywlen  power_dissipated_specify=off  power_dissipated_priority=None  power_dissipated=xgzyrlewkb W  power_dissipated_nominal_specify=off  power_dissipated_nominal_unit=W  power_dissipated_nominal_value=xaufgjttes  thermal_network_parameterization=rhtfzdpkld  Rth=aqkrjbornc K/W  Rth_Foster=cnqtfsutib K/W  thermal_mass_parameterization=xysbimjfwi  thermal_mass=ujjibidbol J/K  thermal_mass_Foster=dehixscchy J/K  thermal_time_constant=prtxkbhlrj s  thermal_time_constant_Foster=tazbjthomj s  thermal_mass_initial_temperatures=qkntalstxl degC
      settings: SourceProductName=Simscape Electrical  InternalSimscapePortConfiguration="{\"Bottom\":[],\"Left\":[{\"id\":\"p\",\"label\":\"\",\"type\":\"foundation.electrical.electrical\"},{\"id\":\"H\",\"label\":\"H\",\"type\":\"foundation.thermal.thermal\"}],\"Right\":[{\"id\":\"n\",\"label\":\"\",\"type\":\"foundation.electrical.electrical\"}],\"Top\":[]}"
  Redacted_7653 : ee_lib/Passive/Thermal/Thermal Resistor  R=tnulhwbazf K/W  T_specify=off  T_priority=None  T=mbqcmvdwox K  T_nominal_specify=off  T_nominal_unit=K  T_nominal_value=ayrbujabnr  Q_specify=off  Q_priority=None  Q=sfclfeggiu W  Q_nominal_specify=off  Q_nominal_unit=W  Q_nominal_value=pymdwgyhnk
      settings: SourceProductName=Simscape Electrical  SourceProductBaseCode=PS  InternalSimscapePortConfiguration="{\"Bottom\":[],\"Left\":[{\"id\":\"A\",\"label\":\"A\",\"type\":\"foundation.thermal.thermal\"}],\"Right\":[{\"id\":\"B\",\"label\":\"B\",\"type\":\"foundation.thermal.thermal\"}],\"Top\":[]}"
  Redacted_9027 : ee_lib/Semiconductors & Converters/Diode  ModelType=jyvxukpdpk  Vf=bdzbpjqkhz V  Ron=lsrjkjootd Ohm  Goff=ofmhtwesaf S  prmExp=bqtdjjwwji  I12=gwyojwxtvw A  V12=tjdwtiqjfm V  IS=pgunbsejse A  ec=gcomlckvkr  I1=iyetrhoopj A  V1=sdybwsehud V  RS=grqlbazvzm Ohm  Tmeas=ctncekrqyd degC  N_series=lxcnowzijw  N_parallel=kurybpjfoc  Rz=txvsbexxwk Ohm  BV=qqelmgxeqk V  C_param=zurgtvxcpf  CJ=nwcsymntkb pF  CJ0=qrfdvnulrv pF  VJ=mgmovfuewc V  Mgrad=ylqxslmpro  Vvec=afcdrhtwnp V  Cvec=gvbmqiulel pF  FC=xunkludvda  Q_param=kbqdjuiass  iRM=rpckqftvfb A  iF=sfeexggdhz A  didt=shdkxcjxfv A/us  trr_factor=jwvirxkxqn  trr=ftzljhgcnc ns  Qrr=upgxindely s*uA  TT=gisgyovfed ns  tau=oqxondjpzp ns  T_param=twxwcrqyec  IS_T2=yfadtlfwty A  I1_T2=yggssgboom A  V1_T2=utgekkynuc V  Tmeas2=osyodgdjlq degC  EG_param=qlkmxtofme  EG=idmsvcfrui eV  XTI_param=toxygxrvnh  XTI=iqhrhfuotd  dBVdT=rgeumoszgp V/K  Tdevice=ffqcgjdiix degC  i_specify=off  i_priority=None  i=bvvibiwhbr A  i_nominal_specify=off  i_nominal_unit=A  i_nominal_value=mnunjczkoc  v_specify=off  v_priority=None  v=zmmshkmtap V  v_nominal_specify=off  v_nominal_unit=V  v_nominal_value=sxmikghxbz  i_capacitor_specify=off  i_capacitor_priority=None  i_capacitor=hcljvkrkqs A  i_capacitor_nominal_specify=off  i_capacitor_nominal_unit=A  i_capacitor_nominal_value=csfodcmgpw  v_capacitor_specify=off  v_capacitor_priority=None  v_capacitor=lettjcqhzu V  v_capacitor_nominal_specify=off  v_capacitor_nominal_unit=V  v_capacitor_nominal_value=fmknydcgsh  power_dissipated_specify=off  power_dissipated_priority=None  power_dissipated=cmvyfkkapt W  power_dissipated_nominal_specify=off  power_dissipated_nominal_unit=W  power_dissipated_nominal_value=gwrobtedsy  thermal_network_parameterization=eykjzgpdvd  Rth=owkxttcwsg K/W  Rth_Foster=lhrazsinzy K/W  thermal_mass_parameterization=rnjojqvdyx  thermal_mass=omrqgtmzbh J/K  thermal_mass_Foster=agkrdtsffb J/K  thermal_time_constant=oqcaefzlvx s  thermal_time_constant_Foster=zpwspxdrsh s  thermal_mass_initial_temperatures=ksvqxybetb degC
      settings: SourceProductName=Simscape Electrical  InternalSimscapePortConfiguration="{\"Bottom\":[],\"Left\":[{\"id\":\"p\",\"label\":\"\",\"type\":\"foundation.electrical.electrical\"},{\"id\":\"H\",\"label\":\"H\",\"type\":\"foundation.thermal.thermal\"}],\"Right\":[{\"id\":\"n\",\"label\":\"\",\"type\":\"foundation.electrical.electrical\"}],\"Top\":[]}"
  Redacted_7604 : PMIOPort  Side=Left
  Redacted_7317 : PMIOPort  Port=2  Side=Left
  Redacted_2449 : PMIOPort  Port=3  Side=Right
  Redacted_1058 : PMIOPort  Port=4  Side=Right
  Redacted_1722 : PMIOPort  Port=5  Side=Left
  Redacted_8069 : PMIOPort  Port=6  Side=Right
  connections:
  Redacted_6160/LConn2 -- Redacted_4934/LConn1
  Redacted_7653/RConn1 -- Redacted_1722/RConn1
  Redacted_1058/RConn1 -- Redacted_2562/RConn2
  Redacted_4076/RConn1 -- Redacted_2562/RConn1 -- Redacted_8069/RConn1
  Redacted_2183/RConn1 -- Redacted_7653/LConn1 -- Redacted_4934/RConn1
  Redacted_7604/RConn1 -- Redacted_9027/RConn1
  Redacted_9027/LConn1 -- Redacted_4076/LConn1
  Redacted_2449/RConn1 -- Redacted_4076/RConn2
  Redacted_9027/LConn2 -- Redacted_2183/LConn1
  Redacted_6160/RConn1 -- Redacted_2562/LConn1
  Redacted_6160/LConn1 -- Redacted_7317/RConn1
